simulink model "VSM_Testcase_Gen_harness"  (R2022a)
settings: Solver=FixedStepDiscrete  StartTime=0  StopTime=0.060000000000000005  FixedStep=0.01  RelTol=1e-3
PostLoadFcn:
  | Sldv.HarnessUtils.openMultiSimulationDesignStudy;
libraries: SignalEditorBlockLib x1, simulink x1
settings Model: DataDictionary=VSM_Data_Dictionary.sldd  EnableAccessToBaseWorkspace=off  SldvGeneratedHarnessModel=TestUnitModel=Vehicle_Speedometer_Module|  Creator=jamesbond  LastModifiedBy=jamesbond
settings OptimizationCC: BlockReduction=off  DefaultParameterBehavior=Inlined  EnhancedBackFolding=on  ExpressionFolding=off  PassReuseOutputArgsAs=Individual arguments  ZeroExternalMemoryAtStartup=off  ZeroInternalMemoryAtStartup=off  OptimizeBlockOrder=speed  DifferentSizesBufferReuse=on  EfficientTunableParamExpr=on
settings DebuggingCC: SignalInfNanChecking=error  SignalRangeChecking=warning  InheritedTsInSrcMsg=none  CheckMatrixSingularityMsg=error  IntegerOverflowMsg=none  ParameterOverflowMsg=none  ParameterTunabilityLossMsg=error  ModelReferenceVersionMismatchMessage=warning  ModelReferenceIOMismatchMessage=warning  IntegerSaturationMsg=none
settings HardwareCC: ProdBitPerLong=64  ProdHWDeviceType=Intel->x86-64 (Mac OS X)
settings SFSimCC: MATLABDynamicMemAlloc=off
settings RTWCC: SystemTargetFile=ert.tlc  GenCodeOnly=on  TemplateMakefile=ert_default_tmf  GenerateReport=on  LaunchReport=on  GenerateCodeMetricsReport=on
settings CodeAppCC: ForceParamTrailComments=on  IgnoreCustomStorageClasses=off  OperatorAnnotations=on  SimulinkDataObjDesc=on  SFDataObjDesc=on  InsertBlockDesc=on
settings ERTTargetCC: TargetLangStandard=C99 (ISO)  GenerateSampleERTMain=on  InlinedParameterPlacement=NonHierarchical  ERTCustomFileTemplate=example_file_process.tlc
settings ConfigComp: CovScope=ReferencedModels  CovIncludeTopModel=off  CovMetricSettings=dcmoe  CovHTMLOptions=-aTS=1 -bRG=1 -bTC=0 -hTR=0 -nFC=0 -scm=1 -bcm=1  DVMaxProcessTime=3000  DVModelCoverageObjectives=MCDC  DVTestSuiteOptimization=Auto  DVDetectDeadLogic=on  DVDetectOutOfBounds=on  DVModelReferenceHarness=on  DVHarnessSource=Signal Editor

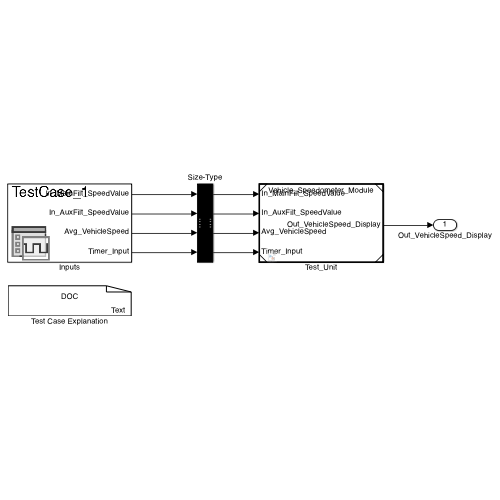
[thumbnail: Simulink's stored preview of the top-level diagram]
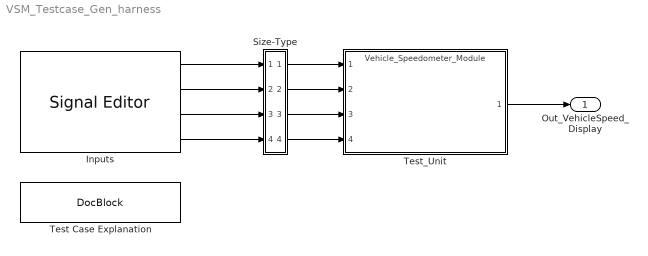
== system VSM_Testcase_Gen_harness ==
  Inputs : SignalEditorBlockLib/Signal Editor  Tag=SignalEditorBlock  FileName=/Users/jamesbond/Desktop/sldv_output/Vehicle_Speedometer_Module/Vehicle_Speedometer_Module_harness_HarnessInputs.mat  ActiveScenario=TestCase_1  ActiveSignal=Timer_Input  IsBus=off  OutputBusObjectStr=Bus: BusObject  SampleTime=[0.01,0]  Interpolate=off  ZeroCross=off  OutputAfterFinalValue=Holding final value  Unit=inherit  PreserveSignalName=off
  Size-Type : Subsystem
  Test Case Explanation : simulink/Model-Wide Utilities/DocBlock  DocumentType=Text
      content=|
      | Test Case 1 (14 Objectives)
      | 	Parameter values:
      |
      | 	1. Speedometer_Module/Input_Processing/Saturation - input >= lower limit true @ T=0.02
      | 	2. Speedometer_Module/Input_Processing/Saturation - input >= lower limit false @ T=0.00
      | 	3. Speedometer_Module/Input_Processing/Saturation - input > upper limit true @ T=0.03
      | 	4. Speedometer_Module/Input_Processing/Saturation - input > upper limit false @ T=0.00
      | 	5. Speedometer_Module/Compare To Zero/Compare - RelationalOperator: input1 == input2 true @ T=0.01
      | 	6. Speedometer_Module/Compare To Zero/Compare - RelationalOperator: input1 == input2 false @ T=0.00
      | 	7. Speedometer_Module/Main_Data_Filtering - Enable control activated true @ T=0.01
      | 	8. Speedometer_Module/Main_Data_Filtering - Enable control activated false @ T=0.00
      | 	9. Speedometer_Module/Auxilliary_Data_Filtering - Enable control activated true @ T=0.01
      | 	10. Speedometer_Module/Auxilliary_Data_Filtering - Enable control activated false @ T=0.00
      | 	11. Speedometer_Module/Display_Speed_Output/Abs - input < 0 true @ T=0.00
      | 	12. Speedometer_Module/Display_Speed_Output/Abs - input < 0 false @ T=0.05
      | 	13. Speedometer_Module/Display_Speed_Output/Relational Operator - RelationalOperator: input1 > input2 true @ T=0.00
      | 	14. Speedometer_Module/Display_Speed_Output/Switch - logical trigger input true (output is from 1st input port) @ T=0.00
      |
      | Test Case 2 (2 Objectives)
      | 	Parameter values:
      |
      | 	1. Speedometer_Module/Display_Speed_Output/Relational Operator - RelationalOperator: input1 > input2 false @ T=0.00
      | 	2. Speedometer_Module/Display_Speed_Output/Switch - logical trigger input false (output is from 3rd input port) @ T=0.00
  Test_Unit : ModelReference  ModelNameDialog=Vehicle_Speedometer_Module  SimulationMode=Normal  ModelReferenceVersion=1.41
  Out_VehicleSpeed_Display : Outport  RequirementInfo={} %GIDa_b4bf2081_ccbe_4f14_8543_6ce2af7ff1ac
  wires:
  Inputs/1 -> Size-Type/1(In1)
  Inputs/2 -> Size-Type/2(In2)
  Inputs/3 -> Size-Type/3(In3)
  Inputs/4 -> Size-Type/4(In4)
  Size-Type/1(Out1) -> Test_Unit/1
  Size-Type/2(Out2) -> Test_Unit/2
  Size-Type/3(Out3) -> Test_Unit/3
  Size-Type/4(Out4) -> Test_Unit/4
  Test_Unit/1 -> Out_VehicleSpeed_Display/1

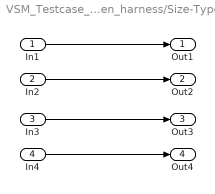
== system VSM_Testcase_Gen_harness/Size-Type ==
  In1 : Inport
  In2 : Inport  Port=2
  In3 : Inport  Port=3
  In4 : Inport  Port=4
  Out1 : Outport
  Out2 : Outport  Port=2
  Out3 : Outport  Port=3
  Out4 : Outport  Port=4
  wires:
  In1/1 -> Out1/1
  In2/1 -> Out2/1
  In3/1 -> Out3/1
  In4/1 -> Out4/1
